simulink model "ModeloCorrea_Cinematico"  (R2023b)
settings: Solver=ode23  StartTime=0.0  StopTime=30  RelTol=1e-3
PreLoadFcn:
  | cargar_datos
model workspace: external: MATLAB File Data\Ensamblaje_Correa_v2_DataFile.m (data not in the file)
undefined symbols (not defined in the file): D, DiscIntNeverNeededParam, Floor, L, R, smiData, X, Y, Z
libraries: sm_lib x464, nesl_utility x23, simulink x8, fl_lib x8, SignalEditorBlockLib x1
(part 1 of 10)
settings Model: Creator=marco  LastModifiedBy=pablo
settings ExplorerConfigSet: InternalSimMechanicsExplorerSettings="<ExplorerConfiguration><canonicalview>default</canonicalview><AnimationSetting><BasePlaybackSpeed>1.0</BasePlaybackSpeed><PlaybackSpeedFactor>1.0</PlaybackSpeedFactor></AnimationSetting><TilePanel><TileInfo><Tiles Columns=\"1\" Count=\"1\" Rows=\"1\"><Column Weight=\"1\"/><Row Weight=\"1\"/><Tile Height=\"1\" Width=\"1\" X=\"0\" Y=\"0\"/></Tiles></TileInfo><SceneInfo><SceneViewer><BGColor><R>0.60000002384185791</R><G>0.60000002384185791</G><B>0.60000002384185791</B></BGColor><Camera><DoPerspective>on</DoPerspective><Position><X>3.93456182089521178</X><Y>0.00766523810611929868</Y><Z>0.735437752381419729</Z></Position><Center><X>3.922559944947976</X><Y>1.61665270142100193</Y><Z>0.0943330044117247912</Z></Center><Up><X>-0.155681862139708971</X><Y>-0.2409665214320105</Y><Z>0.957965705727333972</Z></Up><ViewLimDist>1</ViewLimDist><YLim>0.466307658154998583</YLim><XLim>0.725911711539609095</XLim></Camera></SceneViewer></SceneInfo></TilePanel><MechEditorPanel><Cameras><Camera><Id>Camera1</Id><Value><Name>Camera Esquina</Name><NativeCamera><PositionTrackingFeature>Camaras.Camara_Esquina_Posicion.R</PositionTrackingFeature><CenterTrackingFeature>Camaras.Camara_Aim.R</CenterTrackingFeature><UpVectorTrackingFeature>Camaras.Camara_Esquina_Transformacion.B</UpVectorTrackingFeature><CenterTrackingOrigin>on</CenterTrackingOrigin><UpVectorTrackingDirection>+Z</UpVectorTrackingDirection></NativeCamera></Value></Camera><Camera><Id>Camera2</Id><Value><Name>Camera Lateral</Name><NativeCamera><PositionTrackingFeature>Camaras.Camara_Lateral_Posicion.R</PositionTrackingFeature><CenterTrackingFeature>Camaras.Camara_Aim.R</CenterTrackingFeature><UpVectorTrackingFeature>Camaras.Camara_Lateral_Transformacion.B</UpVectorTrackingFeature><CenterTrackingOrigin>on</CenterTrackingOrigin><UpVectorTrackingDirection>-Y</UpVectorTrackingDirection></NativeCamera></Value></Camera><Camera><Id>Camera3</Id><Value><Name>Camera Superior</Name><NativeCamera><PositionTrackingFeature>Camara_Sup.Camara_Superior_Posicion.R</PositionTrackingFeature><CenterTrackingFeature>Camara_Sup.Camara_Aim.R</CenterTrackingFeature><UpVectorTrackingFeature>Camara_Sup.Camara_Superior_Transformacion.F</UpVectorTrackingFeature><CenterTrackingOrigin>on</CenterTrackingOrigin><UpVectorTrackingDirection>+X</UpVectorTrackingDirection></NativeCamera></Value></Camera></Cameras><GfxPanelCameraMap><MapElement CameraMLId=\"Camera1\" GfxPanelIndex=\"0\"/></GfxPanelCameraMap><VideoCreator><PlaybackSpeedRatio>1.0</PlaybackSpeedRatio><FrameRate>30</FrameRate><VideoFormat>Motion JPEG AVI</VideoFormat><FrameSize>auto</FrameSize></VideoCreator></MechEditorPanel></ExplorerConfiguration>"

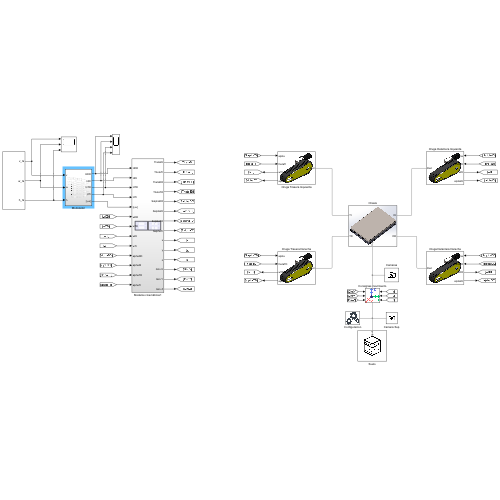
[thumbnail: Simulink's stored preview of the top-level diagram]
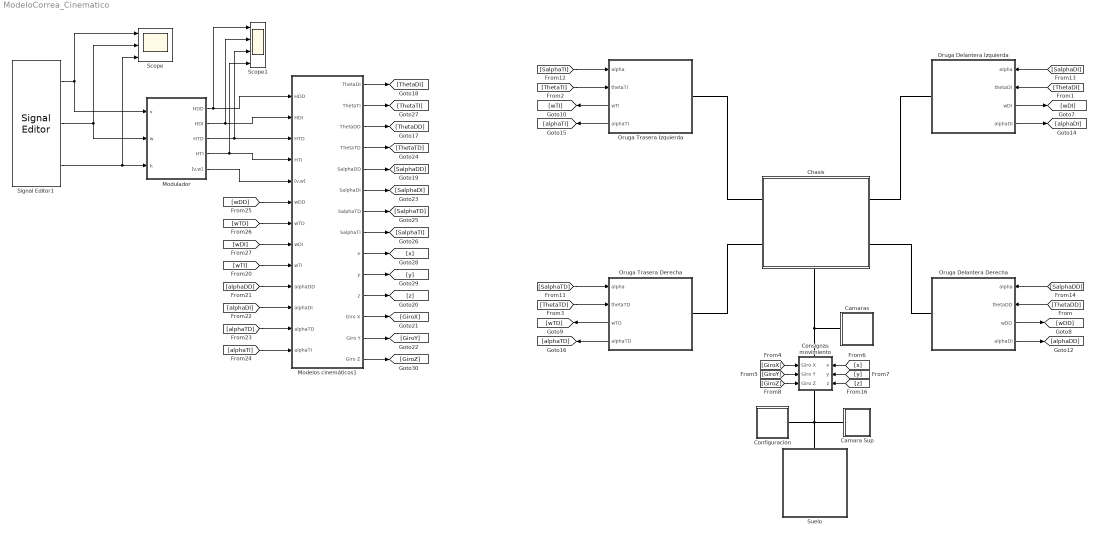
== system ModeloCorrea_Cinematico ==
  Camara Sup : Subsystem
      mask Display: image('photo-camera-icons-photo-camera-icon-design-illustration-photo-camera-simple-sign-photo-camera-logo-free-vector.jpg');
  Camaras : Subsystem
      mask Display: image('photo-camera-icons-photo-camera-icon-design-illustration-photo-camera-simple-sign-photo-camera-logo-free-vector.jpg');
  Chasis : Subsystem
      settings: PortSchema="{\"entries\":[{\"content\":{\"sides\":[{\"content\":{\"connectorIds\":[\"LConn1\",\"LConn2\"]},\"type\":\"ConnectorPlacement.EquallySpacedRectSide\",\"uuid\":\"efc86758-44be-4031-b1cd-a76dbd4a2ab2\"},{\"content\":{\"connectorIds\":[\"RConn1\",\"RConn2\"],\"side\":\"RIGHT\"},\"type\":\"ConnectorPlacement.EquallySpacedRectSide\",\"uuid\":\"c3a2d335-83d2-4f11-a82e-84212a5c33ba\"},{\"content\":{\"side\":\"TOP\"},\"type\":\"ConnectorPlacement.EquallySpacedRectSide\",\"uuid\":\"ad9cdccb-a03b-4b4d-9ef0-e37d712b26c8\"},{\"content\":{\"connectorIds\":[\"RConn3\"],\"side\":\"BOTTOM\"},\"type\":\"ConnectorPlacement.EquallySpacedRectSide\",\"uuid\":\"f3b898e7-922a-430d-876f-1d341c160358\"}]},\"type\":\"ConnectorPlacement.EquallySpacedConnector\",\"uuid\":\"67201c38-8ca0-49d9-b554-1a10d9afc937\"}],\"packageUris\":[\"http://schema.mathworks.com/mf0/Connector/R2020b\"],\"version\":\"1.0\"}"
      mask Display: image('Chasis.png');
  Configuracion : Subsystem
      mask Display: image('config_logo.png');
  Consignas movimiento : Subsystem
      settings: PortSchema="{\"entries\":[{\"content\":{\"sides\":[{\"content\":{\"connectorIds\":[\"In1\",\"In2\",\"In3\"]},\"type\":\"ConnectorPlacement.EquallySpacedRectSide\",\"uuid\":\"6f4dacc9-91b7-4b7c-adf8-17f8e72d409f\"},{\"content\":{\"connectorIds\":[\"In4\",\"In5\",\"In6\"],\"side\":\"RIGHT\"},\"type\":\"ConnectorPlacement.EquallySpacedRectSide\",\"uuid\":\"4738979a-9217-40ad-89d7-912983be4ece\"},{\"content\":{\"connectorIds\":[\"LConn1\"],\"side\":\"TOP\"},\"type\":\"ConnectorPlacement.EquallySpacedRectSide\",\"uuid\":\"3e71380e-8ac2-4639-a71e-f5923b7fda65\"},{\"content\":{\"connectorIds\":[\"RConn1\"],\"side\":\"BOTTOM\"},\"type\":\"ConnectorPlacement.EquallySpacedRectSide\",\"uuid\":\"b318c422-65a3-475f-9e06-26d8c5a1eab3\"}]},\"type\":\"ConnectorPlacement.EquallySpacedConnector\",\"uuid\":\"e032681b-f25a-4d65-b739-2911fc3b0713\"}],\"packageUris\":[\"http://schema.mathworks.com/mf0/Connector/R2020b\"],\"version\":\"1.0\"}"
      mask Display: image('12056247.png');
  Modelos cinemáticos1 : Subsystem
  Modulador : Subsystem
  Oruga Delantera Derecha : Subsystem
      settings: PortSchema="{\"entries\":[{\"content\":{\"sides\":[{\"content\":{\"connectorIds\":[\"LConn1\"]},\"type\":\"ConnectorPlacement.EquallySpacedRectSide\",\"uuid\":\"a1295ca0-b7c0-436a-88be-cceedf21e517\"},{\"content\":{\"connectorIds\":[\"In1\",\"In2\",\"Out1\",\"Out2\"],\"side\":\"RIGHT\"},\"type\":\"ConnectorPlacement.EquallySpacedRectSide\",\"uuid\":\"ea9eb1ac-1c17-440b-aac3-8fa76cfe55ec\"},{\"content\":{\"side\":\"TOP\"},\"type\":\"ConnectorPlacement.EquallySpacedRectSide\",\"uuid\":\"ea9ec6ca-5cdc-41ac-8d7c-823a8b28d2a6\"}]},\"type\":\"ConnectorPlacement.EquallySpacedConnector\",\"uuid\":\"e0ebff2e-a023-4859-a608-17c2594749b2\"}],\"packageUris\":[\"http://schema.mathworks.com/mf0/Connector/R2020b\"],\"version\":\"1.0\"}"
      mask Display: image('OrugaCompleta_Correa.png');
  Oruga Delantera Izquierda : Subsystem
      settings: PortSchema="{\"entries\":[{\"content\":{\"sides\":[{\"content\":{\"connectorIds\":[\"LConn1\"]},\"type\":\"ConnectorPlacement.EquallySpacedRectSide\",\"uuid\":\"a1295ca0-b7c0-436a-88be-cceedf21e517\"},{\"content\":{\"connectorIds\":[\"In1\",\"In2\",\"Out1\",\"Out2\"],\"side\":\"RIGHT\"},\"type\":\"ConnectorPlacement.EquallySpacedRectSide\",\"uuid\":\"ea9eb1ac-1c17-440b-aac3-8fa76cfe55ec\"},{\"content\":{\"side\":\"TOP\"},\"type\":\"ConnectorPlacement.EquallySpacedRectSide\",\"uuid\":\"ea9ec6ca-5cdc-41ac-8d7c-823a8b28d2a6\"}]},\"type\":\"ConnectorPlacement.EquallySpacedConnector\",\"uuid\":\"e0ebff2e-a023-4859-a608-17c2594749b2\"}],\"packageUris\":[\"http://schema.mathworks.com/mf0/Connector/R2020b\"],\"version\":\"1.0\"}"
      mask Display: image('OrugaCompleta_Correa.png');
  Oruga Trasera Derecha : Subsystem
      settings: PortSchema="{\"entries\":[{\"content\":{\"sides\":[{\"content\":{\"connectorIds\":[\"LConn1\"]},\"type\":\"ConnectorPlacement.EquallySpacedRectSide\",\"uuid\":\"a1295ca0-b7c0-436a-88be-cceedf21e517\"},{\"content\":{\"connectorIds\":[\"In1\",\"In2\",\"Out1\",\"Out2\"],\"side\":\"RIGHT\"},\"type\":\"ConnectorPlacement.EquallySpacedRectSide\",\"uuid\":\"ea9eb1ac-1c17-440b-aac3-8fa76cfe55ec\"},{\"content\":{\"side\":\"TOP\"},\"type\":\"ConnectorPlacement.EquallySpacedRectSide\",\"uuid\":\"ea9ec6ca-5cdc-41ac-8d7c-823a8b28d2a6\"}]},\"type\":\"ConnectorPlacement.EquallySpacedConnector\",\"uuid\":\"e0ebff2e-a023-4859-a608-17c2594749b2\"}],\"packageUris\":[\"http://schema.mathworks.com/mf0/Connector/R2020b\"],\"version\":\"1.0\"}"
      mask Display: image('OrugaCompleta_Correa.png');
  Oruga Trasera Izquierda : Subsystem
      settings: PortSchema="{\"entries\":[{\"content\":{\"sides\":[{\"content\":{\"connectorIds\":[\"LConn1\"]},\"type\":\"ConnectorPlacement.EquallySpacedRectSide\",\"uuid\":\"a1295ca0-b7c0-436a-88be-cceedf21e517\"},{\"content\":{\"connectorIds\":[\"In1\",\"In2\",\"Out1\",\"Out2\"],\"side\":\"RIGHT\"},\"type\":\"ConnectorPlacement.EquallySpacedRectSide\",\"uuid\":\"ea9eb1ac-1c17-440b-aac3-8fa76cfe55ec\"},{\"content\":{\"side\":\"TOP\"},\"type\":\"ConnectorPlacement.EquallySpacedRectSide\",\"uuid\":\"ea9ec6ca-5cdc-41ac-8d7c-823a8b28d2a6\"}]},\"type\":\"ConnectorPlacement.EquallySpacedConnector\",\"uuid\":\"e0ebff2e-a023-4859-a608-17c2594749b2\"}],\"packageUris\":[\"http://schema.mathworks.com/mf0/Connector/R2020b\"],\"version\":\"1.0\"}"
      mask Display: image('OrugaCompleta_Correa.png');
  Scope : Scope  NumInputPorts=3
  Scope1 : Scope  NumInputPorts=4
  Signal Editor1 : SignalEditorBlockLib/Signal Editor  FileName=datos_modelo.mat  ActiveScenario=modelo  ActiveSignal=v_ts  IsBus=off  OutputBusObjectStr=Bus: BusObject  SampleTime=0.1  ZeroCross=off  OutputAfterFinalValue=Setting to zero  Unit=inherit  PreserveSignalName=on  ApplySigPropsToAllScenarios=on  ApplySigPropsToAllSignals=on
  Suelo : Subsystem
      mask Display: image('suelo_icon.jpg');
  wires:
  [ThetaDD] -> Oruga Delantera Derecha/2(thetaDD)
  [ThetaDI] -> Oruga Delantera Izquierda/2(thetaDI)
  [ThetaTI] -> Oruga Trasera Izquierda/2(thetaTI)
  [ThetaTD] -> Oruga Trasera Derecha/2(thetaTD)
  Oruga Delantera Izquierda/1(wDI) -> [wDI]
  Oruga Delantera Derecha/1(wDD) -> [wDD]
  Oruga Trasera Derecha/1(wTD) -> [wTD]
  Oruga Trasera Izquierda/1(wTI) -> [wTI]
  [SalphaTD] -> Oruga Trasera Derecha/1(alpha)
  [SalphaTI] -> Oruga Trasera Izquierda/1(alpha)
  [SalphaDI] -> Oruga Delantera Izquierda/1(alpha)
  [SalphaDD] -> Oruga Delantera Derecha/1(alpha)
  Oruga Delantera Derecha/2(alphaDI) -> [alphaDD]
  Oruga Delantera Izquierda/2(alphaDI) -> [alphaDI]
  Oruga Trasera Izquierda/2(alphaTI) -> [alphaTI]
  Oruga Trasera Derecha/2(alphaTD) -> [alphaTD]
  Modelos cinemáticos1/2(ThetaTI) -> [ThetaTI]
  Modelos cinemáticos1/8(SalphaTI) -> [SalphaTI]
  Modelos cinemáticos1/7(SalphaTD) -> [SalphaTD]
  Modelos cinemáticos1/6(SalphaDI) -> [SalphaDI]
  [wDI] -> Modelos cinemáticos1/8(wDI)
  Modelos cinemáticos1/1(ThetaDI) -> [ThetaDI]
  Modelos cinemáticos1/3(ThetaDD) -> [ThetaDD]
  [alphaTI] -> Modelos cinemáticos1/13(alphaTI)
  Modelos cinemáticos1/5(SalphaDD) -> [SalphaDD]
  Modelos cinemáticos1/4(ThetaTD) -> [ThetaTD]
  Modelos cinemáticos1/10(y) -> [y]
  Modelos cinemáticos1/12(Giro X) -> [GiroX]
  [alphaTD] -> Modelos cinemáticos1/12(alphaTD)
  [alphaDI] -> Modelos cinemáticos1/11(alphaDI)
  Modelos cinemáticos1/9(x) -> [x]
  [alphaDD] -> Modelos cinemáticos1/10(alphaDD)
  [wTI] -> Modelos cinemáticos1/9(wTI)
  [wDD] -> Modelos cinemáticos1/6(wDD)
  Modelos cinemáticos1/14(Giro Z) -> [GiroZ]
  [wTD] -> Modelos cinemáticos1/7(wTD)
  Modelos cinemáticos1/11(z) -> [z]
  Modelos cinemáticos1/13(Giro Y) -> [GiroY]
  [GiroZ] -> Consignas movimiento/3(Giro Z)
  [x] -> Consignas movimiento/4(x)
  [GiroY] -> Consignas movimiento/2(Giro Y)
  [GiroX] -> Consignas movimiento/1(Giro X)
  [z] -> Consignas movimiento/6(z)
  [y] -> Consignas movimiento/5(y)
  Signal Editor1/2 -> Scope/2, Modulador/2(w)
  Signal Editor1/1 -> Scope/1, Modulador/1(v)
  Modulador/1(HDD) -> Scope1/1, Modelos cinemáticos1/1(HDD)
  Modulador/2(HDI) -> Scope1/2, Modelos cinemáticos1/2(HDI)
  Modulador/3(HTD) -> Scope1/3, Modelos cinemáticos1/3(HTD)
  Modulador/4(HTI) -> Modelos cinemáticos1/4(HTI), Scope1/4
  Modulador/5("[v,w]") -> Modelos cinemáticos1/5("[v,w]")
  Signal Editor1/3 -> Modulador/3(h), Scope/3
  connections:
  Suelo/LConn1 -- Camara Sup/RConn1 -- Consignas movimiento/RConn1 -- Configuracion/RConn1
  Chasis/LConn2 -- Oruga Trasera Derecha/LConn1
  Chasis/LConn1 -- Oruga Trasera Izquierda/LConn1
  Chasis/RConn1 -- Oruga Delantera Izquierda/LConn1
  Chasis/RConn2 -- Oruga Delantera Derecha/LConn1
  Camaras/RConn1 -- Chasis/RConn3 -- Consignas movimiento/LConn1

== system ModeloCorrea_Cinematico/Camara Sup ==
  Camara Aim : sm_lib/Frames and Transforms/Reference Frame
  Camara Superior Posicion : sm_lib/Frames and Transforms/Reference Frame
  Camara Superior Transformacion : sm_lib/Frames and Transforms/Rigid Transform  TranslationMethod=Cartesian  TranslationStandardOffset=0  TranslationStandardOffsetUnits=m  TranslationStandardAxis=+Z  TranslationCartesianOffset=[0 0 -10]  TranslationCartesianOffsetUnits=m  TranslationROffset=0  TranslationROffsetUnits=m  TranslationZOffset=0  TranslationZOffsetUnits=m  TranslationThetaOffset=0  TranslationThetaOffsetUnits=deg  RotationMethod=None  RotationAngleUnits=deg  RotationStandardAxis=+Z  RotationAngle=0.0  RotationArbitraryAxis=[0 0 1]  FollAlignAxisA=+X  BaseAlignAxisA=+Y  FollAlignAxisB=+Y  BaseAlignAxisB=+Z  RotationSequenceAxes=FollowerAxes  RotationSequence=XYX  RotationSequenceAngles=[0 0 0]  RotationSequenceAnglesUnits=deg  RotationMatrix=[1 0 0; 0 1 0; 0 0 1]  Quaternion=[1 0 0 0]
  Camara Superior : PMIOPort  Side=Right
  connections:
  Camara Superior Posicion/RConn1 -- Camara Superior Transformacion/LConn1
  Camara Aim/RConn1 -- Camara Superior Transformacion/RConn1 -- Camara Superior/RConn1

== system ModeloCorrea_Cinematico/Camaras ==
  Camara Aim : sm_lib/Frames and Transforms/Reference Frame
  Camara Esquina Posicion : sm_lib/Frames and Transforms/Reference Frame
  Camara Esquina Transformacion : sm_lib/Frames and Transforms/Rigid Transform  TranslationMethod=Cartesian  TranslationStandardOffset=0  TranslationStandardOffsetUnits=m  TranslationStandardAxis=+Z  TranslationCartesianOffset=[-1 -1 -1]  TranslationCartesianOffsetUnits=m  TranslationROffset=0  TranslationROffsetUnits=m  TranslationZOffset=0  TranslationZOffsetUnits=m  TranslationThetaOffset=0  TranslationThetaOffsetUnits=deg  RotationMethod=None  RotationAngleUnits=deg  RotationStandardAxis=+Z  RotationAngle=0.0  RotationArbitraryAxis=[0 0 1]  FollAlignAxisA=+X  BaseAlignAxisA=+Y  FollAlignAxisB=+Y  BaseAlignAxisB=+Z  RotationSequenceAxes=FollowerAxes  RotationSequence=XYX  RotationSequenceAngles=[0 0 0]  RotationSequenceAnglesUnits=deg  RotationMatrix=[1 0 0; 0 1 0; 0 0 1]  Quaternion=[1 0 0 0]
  Camara Lateral Posicion : sm_lib/Frames and Transforms/Reference Frame
  Camara Lateral Transformacion : sm_lib/Frames and Transforms/Rigid Transform  TranslationMethod=Cartesian  TranslationStandardOffset=0  TranslationStandardOffsetUnits=m  TranslationStandardAxis=+Z  TranslationCartesianOffset=[0 -2 -0.30]  TranslationCartesianOffsetUnits=m  TranslationROffset=0  TranslationROffsetUnits=m  TranslationZOffset=0  TranslationZOffsetUnits=m  TranslationThetaOffset=0  TranslationThetaOffsetUnits=deg  RotationMethod=None  RotationAngleUnits=deg  RotationStandardAxis=+Z  RotationAngle=0.0  RotationArbitraryAxis=[0 0 1]  FollAlignAxisA=+X  BaseAlignAxisA=+Y  FollAlignAxisB=+Y  BaseAlignAxisB=+Z  RotationSequenceAxes=FollowerAxes  RotationSequence=XYX  RotationSequenceAngles=[0 0 0]  RotationSequenceAnglesUnits=deg  RotationMatrix=[1 0 0; 0 1 0; 0 0 1]  Quaternion=[1 0 0 0]
  Camaras : PMIOPort  Side=Right
  connections:
  Camara Esquina Transformacion/RConn1 -- Camara Lateral Transformacion/RConn1 -- Camara Aim/RConn1 -- Camaras/RConn1
  Camara Esquina Posicion/RConn1 -- Camara Esquina Transformacion/LConn1
  Camara Lateral Posicion/RConn1 -- Camara Lateral Transformacion/LConn1

== system ModeloCorrea_Cinematico/Chasis ==
  ReferenceFrame : sm_lib/Frames and Transforms/Reference Frame
  Rigid Transform1 : sm_lib/Frames and Transforms/Rigid Transform  TranslationMethod=Cartesian  TranslationStandardOffset=91.5  TranslationStandardOffsetUnits=mm  TranslationStandardAxis=-X  TranslationCartesianOffset=[91.5 -70 +158.5]  TranslationCartesianOffsetUnits=mm  TranslationROffset=0  TranslationROffsetUnits=m  TranslationZOffset=0  TranslationZOffsetUnits=m  TranslationThetaOffset=0  TranslationThetaOffsetUnits=deg  RotationMethod=StandardAxis  RotationAngleUnits=deg  RotationStandardAxis=+Y  RotationAngle=180  RotationArbitraryAxis=[1 1 0]  FollAlignAxisA=+X  BaseAlignAxisA=+Y  FollAlignAxisB=+Y  BaseAlignAxisB=+Z  RotationSequenceAxes=FollowerAxes  RotationSequence=XYX  RotationSequenceAngles=[180 180 0]  RotationSequenceAnglesUnits=deg  RotationMatrix=[0 180 0; 0 1 0; 0 0 1]  Quaternion=[1 0 0 0]
  Rigid Transform2 : sm_lib/Frames and Transforms/Rigid Transform  TranslationMethod=Cartesian  TranslationStandardOffset=91.5  TranslationStandardOffsetUnits=mm  TranslationStandardAxis=-X  TranslationCartesianOffset=[91.5 -70 -158.5]  TranslationCartesianOffsetUnits=mm  TranslationROffset=0  TranslationROffsetUnits=m  TranslationZOffset=0  TranslationZOffsetUnits=m  TranslationThetaOffset=0  TranslationThetaOffsetUnits=deg  RotationMethod=StandardAxis  RotationAngleUnits=deg  RotationStandardAxis=+Y  RotationAngle=180  RotationArbitraryAxis=[0 0 1]  FollAlignAxisA=+X  BaseAlignAxisA=+Y  FollAlignAxisB=+Y  BaseAlignAxisB=+Z  RotationSequenceAxes=FollowerAxes  RotationSequence=XYX  RotationSequenceAngles=[0 0 0]  RotationSequenceAnglesUnits=deg  RotationMatrix=[1 0 0; 0 1 0; 0 0 1]  Quaternion=[1 0 0 0]
  Rigid Transform3 : sm_lib/Frames and Transforms/Rigid Transform  TranslationMethod=Cartesian  TranslationStandardOffset=91.5  TranslationStandardOffsetUnits=mm  TranslationStandardAxis=-X  TranslationCartesianOffset=[-91.5 -70 -158.5]  TranslationCartesianOffsetUnits=mm  TranslationROffset=0  TranslationROffsetUnits=m  TranslationZOffset=0  TranslationZOffsetUnits=m  TranslationThetaOffset=0  TranslationThetaOffsetUnits=deg  RotationMethod=None  RotationAngleUnits=deg  RotationStandardAxis=+X  RotationAngle=180  RotationArbitraryAxis=[1 1 0]  FollAlignAxisA=+X  BaseAlignAxisA=+Y  FollAlignAxisB=+Y  BaseAlignAxisB=+Z  RotationSequenceAxes=FollowerAxes  RotationSequence=XYX  RotationSequenceAngles=[180 180 0]  RotationSequenceAnglesUnits=deg  RotationMatrix=[0 180 0; 0 1 0; 0 0 1]  Quaternion=[1 0 0 0]
  Rigid Transform4 : sm_lib/Frames and Transforms/Rigid Transform  TranslationMethod=Cartesian  TranslationStandardOffset=91.5  TranslationStandardOffsetUnits=mm  TranslationStandardAxis=-X  TranslationCartesianOffset=[-91.5 -70 158.5]  TranslationCartesianOffsetUnits=mm  TranslationROffset=0  TranslationROffsetUnits=m  TranslationZOffset=0  TranslationZOffsetUnits=m  TranslationThetaOffset=0  TranslationThetaOffsetUnits=deg  RotationMethod=None  RotationAngleUnits=deg  RotationStandardAxis=+Z  RotationAngle=0.0  RotationArbitraryAxis=[0 0 1]  FollAlignAxisA=+X  BaseAlignAxisA=+Y  FollAlignAxisB=+Y  BaseAlignAxisB=+Z  RotationSequenceAxes=FollowerAxes  RotationSequence=XYX  RotationSequenceAngles=[0 0 0]  RotationSequenceAnglesUnits=deg  RotationMatrix=[1 0 0; 0 1 0; 0 0 1]  Quaternion=[1 0 0 0]
  Rigid Transform5 : sm_lib/Frames and Transforms/Rigid Transform  TranslationMethod=StandardAxis  TranslationStandardOffset=235  TranslationStandardOffsetUnits=mm  TranslationStandardAxis=+Z  TranslationCartesianOffset=[0 0 0]  TranslationCartesianOffsetUnits=m  TranslationROffset=0  TranslationROffsetUnits=m  TranslationZOffset=0  TranslationZOffsetUnits=m  TranslationThetaOffset=0  TranslationThetaOffsetUnits=deg  RotationMethod=StandardAxis  RotationAngleUnits=deg  RotationStandardAxis=+X  RotationAngle=90  RotationArbitraryAxis=[0 0 1]  FollAlignAxisA=+X  BaseAlignAxisA=+Y  FollAlignAxisB=+Y  BaseAlignAxisB=+Z  RotationSequenceAxes=FollowerAxes  RotationSequence=XYX  RotationSequenceAngles=[0 0 0]  RotationSequenceAnglesUnits=deg  RotationMatrix=[1 0 0; 0 1 0; 0 0 1]  Quaternion=[1 0 0 0]
  Solid : sm_lib/Body Elements/File Solid  ExtGeomFileName=CAD\Chasis.STEP  UnitType=FromFile  ExtGeomFileUnits=m  StepReaderType=HEX  ExportConvexHullGeometry=off  InertiaType=Custom  Mass=100  MassUnits=kg  CenterOfMass=smiData.Solid(19).CoM  CenterOfMassUnits=mm  MomentsOfInertia=smiData.Solid(19).MoI  MomentsOfInertiaUnits=kg*mm^2  ProductsOfInertia=smiData.Solid(19).PoI  ProductsOfInertiaUnits=kg*mm^2  BasedOnType=DensityFromFile  Density=1000  DensityUnits=kg/m^3  DoExposeReferenceFrame=on  SerializedFrames=<Frames/>  GraphicType=FromGeometry  MarkerShape=Sphere  MarkerSize=10  GraphicVisPropType=SimpleVisualProperties  GraphicDiffuseColor=[0.6 0.6 0.6]  GraphicSpecularColor=[0.5 0.5 0.5 1.0]  GraphicAmbientColor=[0.15 0.15 0.15 1.0]  GraphicEmissiveColor=[0.0 0.0 0.0 1.0]  GraphicShininess=75  GraphicOpacity=smiData.Solid(19).opacity
  TI : PMIOPort  Side=Left
  TD : PMIOPort  Port=2  Side=Left
  DI : PMIOPort  Port=3  Side=Right
  DD : PMIOPort  Port=4  Side=Right
  Input : PMIOPort  Port=5  Side=Right
  connections:
  Rigid Transform5/LConn1 -- Input/RConn1
  TD/RConn1 -- Rigid Transform4/RConn1
  Rigid Transform3/LConn1 -- Rigid Transform2/LConn1 -- Solid/RConn1 -- Rigid Transform1/LConn1 -- Rigid Transform5/RConn1 -- Rigid Transform4/LConn1 -- ReferenceFrame/RConn1
  Rigid Transform3/RConn1 -- TI/RConn1
  DI/RConn1 -- Rigid Transform2/RConn1
  Rigid Transform1/RConn1 -- DD/RConn1

== system ModeloCorrea_Cinematico/Configuracion ==
  MechanismConfiguration : sm_lib/Utilities/Mechanism Configuration  UniformGravity=Constant  GravityVector=[0 -9.80665 0]  GravityVectorUnits=m/s^2  LinearizationDelta=0.001  JointModeTransitionNonlinearIterations=2
  Solver Configuration : nesl_utility/Solver Configuration  PhysicalDomain=network_engine_domain  SubClassName=solver  LeftPortType=input  RightPortType=generic  Tones=[]  Harmonics=[]  SimulateNoise=off  Profile=off  UseLocalSampling=off  EnableSwitchedLinearOptims=on  FrequencyDomain=off  UseCCode=off  RelTol=0.001  AbsTol=0.001  MinStep=1e-09  ToWorkspace=off  RevertToSquareIcSolve=off  NumHomotopyIterations=100  PhasorMode=off  PhasorModeNumHarmonics=1  ConsistencySolver=NEWTON_XTOL_AFTER_FTOL  IndexReductionMethod=DerivativeReplacement  DoDC=off  ResidualTolerance=1e-09  ConsistencyTolSource=GLOBAL  ConsistencyAbsTol=0.001  ConsistencyRelTol=0.001  ConsistencyTolFactor=0.001  UseLocalSolver=off  LocalSolverChoice=NE_BACKWARD_EULER_ADVANCER  ResolveIndetEquations=on  FunctionEvalNumThread=1  LocalSolverSampleTime=0.001  DoFixedCost=off  MaxNonlinIter=3  MaxModeIter=2  ComputeImpulses=off  ImpulseIterations=2  LinearAlgebra=auto  LinearAlgebraNumThread=0  EquationFormulation=NE_TIME_EF  DelaysMemoryBudget=1024  AutomaticFiltering=on  FilteringTimeConstant=0.001  PartitionStorageMethod=AS_NEEDED  PartitionMemoryBudget=1024  PartitionMethod=ROBUST  MultibodyUseLocalSolver=off  MultibodyLocalSolverChoice=ODE1  MultibodyLocalSolverSampleTime=0.001
  World : sm_lib/Frames and Transforms/World Frame
  a : PMIOPort  Side=Right
  connections:
  World/RConn1 -- MechanismConfiguration/RConn1 -- Solver Configuration/RConn1 -- a/RConn1

== system ModeloCorrea_Cinematico/Consignas movimiento ==
  Giro X : Inport
  Giro Y : Inport  Port=2
  Giro Z : Inport  Port=3
  x : Inport  Port=4
  y : Inport  Port=5
  z : Inport  Port=6
  Bushing Joint : sm_lib/Joints/Bushing Joint  JointMode=Normal  SenseConstraintForce=off  SenseConstraintForceX=off  SenseConstraintForceY=off  SenseConstraintForceZ=off  SenseConstraintTorque=off  SenseConstraintTorqueX=off  SenseConstraintTorqueY=off  SenseConstraintTorqueZ=off  SenseTotalForce=off  SenseTotalForceX=off  SenseTotalForceY=off  SenseTotalForceZ=off  SenseTotalTorque=off  SenseTotalTorqueX=off  SenseTotalTorqueY=off  SenseTotalTorqueZ=off  CompositeWrenchDir=BaseOnFollower  CompositeWrenchFrame=BaseFrame  PxEquilibriumPosition=0  PxEquilibriumPositionUnits=m  PxSpringStiffness=0  PxSpringStiffnessUnits=N/m  PxDampingCoefficient=0  PxDampingCoefficientUnits=N/(m/s)  PxTorqueActuationMode=ComputedTorque  PxMotionActuationMode=InputMotion  PxSensePosition=off  PxSenseVelocity=off  PxSenseAcceleration=off  PxSenseTorqueForce=off  PxSenseLowerLimitTorqueForce=off  PxSenseUpperLimitTorqueForce=off  PxLowerLimitSpecify=off  PxLowerLimitBound=-1  PxLowerLimitBoundUnits=m  PxLowerLimitStiffness=1e6  PxLowerLimitStiffnessUnits=N/m  PxLowerLimitDamping=1e3  PxLowerLimitDampingUnits=N/(m/s)  PxLowerLimitTransitionRegionWidth=1e-4  PxLowerLimitTransitionRegionWidthUnits=m  PxUpperLimitSpecify=off  PxUpperLimitBound=1  PxUpperLimitBoundUnits=m  PxUpperLimitStiffness=1e6  PxUpperLimitStiffnessUnits=N/m  PxUpperLimitDamping=1e3  PxUpperLimitDampingUnits=N/(m/s)  PxUpperLimitTransitionRegionWidth=1e-4  PxUpperLimitTransitionRegionWidthUnits=m  PxPositionTargetSpecify=off  PxPositionTargetPriority=High  PxPositionTargetValue=0  PxPositionTargetValueUnits=m  PxVelocityTargetSpecify=off  PxVelocityTargetPriority=High  PxVelocityTargetValue=0  PxVelocityTargetValueUnits=m/s  PyEquilibriumPosition=0  PyEquilibriumPositionUnits=m  PySpringStiffness=0  PySpringStiffnessUnits=N/m  PyDampingCoefficient=0  PyDampingCoefficientUnits=N/(m/s)  PyTorqueActuationMode=ComputedTorque  PyMotionActuationMode=InputMotion  PySensePosition=off  PySenseVelocity=off  PySenseAcceleration=off  PySenseTorqueForce=off  PySenseLowerLimitTorqueForce=off  PySenseUpperLimitTorqueForce=off  PyLowerLimitSpecify=off  PyLowerLimitBound=-1  PyLowerLimitBoundUnits=m  PyLowerLimitStiffness=1e6  PyLowerLimitStiffnessUnits=N/m  PyLowerLimitDamping=1e3  PyLowerLimitDampingUnits=N/(m/s)  PyLowerLimitTransitionRegionWidth=1e-4  PyLowerLimitTransitionRegionWidthUnits=m  PyUpperLimitSpecify=off  PyUpperLimitBound=1  PyUpperLimitBoundUnits=m  PyUpperLimitStiffness=1e6  PyUpperLimitStiffnessUnits=N/m  PyUpperLimitDamping=1e3  PyUpperLimitDampingUnits=N/(m/s)  PyUpperLimitTransitionRegionWidth=1e-4  PyUpperLimitTransitionRegionWidthUnits=m  PyPositionTargetSpecify=off  PyPositionTargetPriority=High  PyPositionTargetValue=0  PyPositionTargetValueUnits=m  PyVelocityTargetSpecify=off  PyVelocityTargetPriority=High  PyVelocityTargetValue=0  PyVelocityTargetValueUnits=m/s  PzEquilibriumPosition=0  PzEquilibriumPositionUnits=m  PzSpringStiffness=0  PzSpringStiffnessUnits=N/m  PzDampingCoefficient=0  PzDampingCoefficientUnits=N/(m/s)  PzTorqueActuationMode=ComputedTorque  PzMotionActuationMode=InputMotion  PzSensePosition=off  PzSenseVelocity=off  PzSenseAcceleration=off  PzSenseTorqueForce=off  PzSenseLowerLimitTorqueForce=off  PzSenseUpperLimitTorqueForce=off  PzLowerLimitSpecify=off  PzLowerLimitBound=-1  PzLowerLimitBoundUnits=m  PzLowerLimitStiffness=1e6  PzLowerLimitStiffnessUnits=N/m  PzLowerLimitDamping=1e3  PzLowerLimitDampingUnits=N/(m/s)  PzLowerLimitTransitionRegionWidth=1e-4  PzLowerLimitTransitionRegionWidthUnits=m  PzUpperLimitSpecify=off  PzUpperLimitBound=1  PzUpperLimitBoundUnits=m  PzUpperLimitStiffness=1e6  PzUpperLimitStiffnessUnits=N/m  PzUpperLimitDamping=1e3  PzUpperLimitDampingUnits=N/(m/s)  PzUpperLimitTransitionRegionWidth=1e-4  PzUpperLimitTransitionRegionWidthUnits=m  PzPositionTargetSpecify=off  PzPositionTargetPriority=High  PzPositionTargetValue=0  PzPositionTargetValueUnits=m  PzVelocityTargetSpecify=off  PzVelocityTargetPriority=High  PzVelocityTargetValue=0  PzVelocityTargetValueUnits=m/s  RxEquilibriumPosition=0  RxEquilibriumPositionUnits=deg  RxSpringStiffness=0  RxSpringStiffnessUnits=N*m/deg  RxDampingCoefficient=0  RxDampingCoefficientUnits=N*m/(deg/s)  RxTorqueActuationMode=ComputedTorque  RxMotionActuationMode=InputMotion  RxSensePosition=off  RxSenseVelocity=off  RxSenseAcceleration=off  RxSenseTorqueForce=off  RxSenseLowerLimitTorqueForce=off  RxSenseUpperLimitTorqueForce=off  RxLowerLimitSpecify=off  RxLowerLimitBound=-90  RxLowerLimitBoundUnits=deg  RxLowerLimitStiffness=1e4  RxLowerLimitStiffnessUnits=N*m/deg  RxLowerLimitDamping=10  RxLowerLimitDampingUnits=N*m/(deg/s)  RxLowerLimitTransitionRegionWidth=0.1  RxLowerLimitTransitionRegionWidthUnits=deg  RxUpperLimitSpecify=off  RxUpperLimitBound=90  RxUpperLimitBoundUnits=deg  RxUpperLimitStiffness=1e4  RxUpperLimitStiffnessUnits=N*m/deg  RxUpperLimitDamping=10  RxUpperLimitDampingUnits=N*m/(deg/s)  RxUpperLimitTransitionRegionWidth=0.1  RxUpperLimitTransitionRegionWidthUnits=deg  RxPositionTargetSpecify=off  RxPositionTargetPriority=High  RxPositionTargetValue=0  RxPositionTargetValueUnits=deg  RxVelocityTargetSpecify=off  RxVelocityTargetPriority=High  RxVelocityTargetValue=0  RxVelocityTargetValueUnits=deg/s  RyEquilibriumPosition=0  RyEquilibriumPositionUnits=deg  RySpringStiffness=0  RySpringStiffnessUnits=N*m/deg  RyDampingCoefficient=0  RyDampingCoefficientUnits=N*m/(deg/s)  RyTorqueActuationMode=ComputedTorque  RyMotionActuationMode=InputMotion  RySensePosition=off  RySenseVelocity=off  RySenseAcceleration=off  RySenseTorqueForce=off  RySenseLowerLimitTorqueForce=off  RySenseUpperLimitTorqueForce=off  RyLowerLimitSpecify=off  RyLowerLimitBound=-90  RyLowerLimitBoundUnits=deg  RyLowerLimitStiffness=1e4  RyLowerLimitStiffnessUnits=N*m/deg  RyLowerLimitDamping=10  RyLowerLimitDampingUnits=N*m/(deg/s)  RyLowerLimitTransitionRegionWidth=0.1  RyLowerLimitTransitionRegionWidthUnits=deg  RyUpperLimitSpecify=off  RyUpperLimitBound=90  RyUpperLimitBoundUnits=deg  RyUpperLimitStiffness=1e4  RyUpperLimitStiffnessUnits=N*m/deg  RyUpperLimitDamping=10  RyUpperLimitDampingUnits=N*m/(deg/s)  RyUpperLimitTransitionRegionWidth=0.1  RyUpperLimitTransitionRegionWidthUnits=deg  RyPositionTargetSpecify=off  RyPositionTargetPriority=High  RyPositionTargetValue=0  RyPositionTargetValueUnits=deg  RyVelocityTargetSpecify=off  RyVelocityTargetPriority=High  RyVelocityTargetValue=0  RyVelocityTargetValueUnits=deg/s  RzEquilibriumPosition=0  RzEquilibriumPositionUnits=deg  RzSpringStiffness=0  RzSpringStiffnessUnits=N*m/deg  RzDampingCoefficient=0  RzDampingCoefficientUnits=N*m/(deg/s)  RzTorqueActuationMode=ComputedTorque  RzMotionActuationMode=InputMotion  RzSensePosition=off  RzSenseVelocity=off  RzSenseAcceleration=off  RzSenseTorqueForce=off  RzSenseLowerLimitTorqueForce=off  RzSenseUpperLimitTorqueForce=off  RzLowerLimitSpecify=off  RzLowerLimitBound=-90  RzLowerLimitBoundUnits=deg  RzLowerLimitStiffness=1e4  RzLowerLimitStiffnessUnits=N*m/deg  RzLowerLimitDamping=10  RzLowerLimitDampingUnits=N*m/(deg/s)  RzLowerLimitTransitionRegionWidth=0.1  RzLowerLimitTransitionRegionWidthUnits=deg  RzUpperLimitSpecify=off  RzUpperLimitBound=90  RzUpperLimitBoundUnits=deg  RzUpperLimitStiffness=1e4  RzUpperLimitStiffnessUnits=N*m/deg  RzUpperLimitDamping=10  RzUpperLimitDampingUnits=N*m/(deg/s)  RzUpperLimitTransitionRegionWidth=0.1  RzUpperLimitTransitionRegionWidthUnits=deg  RzPositionTargetSpecify=off  RzPositionTargetPriority=High  RzPositionTargetValue=0  RzPositionTargetValueUnits=deg  RzVelocityTargetSpecify=off  RzVelocityTargetPriority=High  RzVelocityTargetValue=0  RzVelocityTargetValueUnits=deg/s
  Simulink-PS Converter{,1..5} (6 alike) : nesl_utility/Simulink-PS Converter  PhysicalDomain=network_engine_domain  SubClassName=ps_input  LeftPortType=input  RightPortType=output  PseudoPeriodic=off  Frequencies=[]  NoiseDistribution=none  NoiseParameters=[]  Unit=1  AffineConversion=off  FilteringAndDerivatives=filter  SimscapeFilterOrder=2  InputFilterTimeConstant=0.001  UdotUserProvided=0
  Output : PMIOPort  Side=Left
  Input : PMIOPort  Port=2  Side=Right
  wires:
  Giro Z/1 -> Simulink-PS Converter4/1
  x/1 -> Simulink-PS Converter/1
  y/1 -> Simulink-PS Converter1/1
  Giro X/1 -> Simulink-PS Converter3/1
  Giro Y/1 -> Simulink-PS Converter5/1
  z/1 -> Simulink-PS Converter2/1
  connections:
  Bushing Joint/RConn1 -- Output/RConn1
  Bushing Joint/LConn1 -- Input/RConn1
  Simulink-PS Converter/RConn1 -- Bushing Joint/LConn2
  Simulink-PS Converter1/RConn1 -- Bushing Joint/LConn3
  Simulink-PS Converter2/RConn1 -- Bushing Joint/LConn4
  Simulink-PS Converter3/RConn1 -- Bushing Joint/LConn5
  Simulink-PS Converter5/RConn1 -- Bushing Joint/LConn6
  Simulink-PS Converter4/RConn1 -- Bushing Joint/LConn7

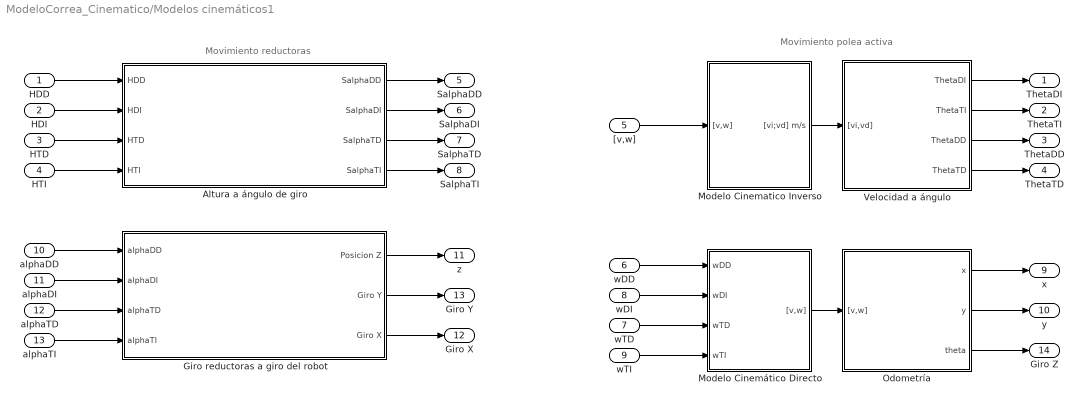
== system ModeloCorrea_Cinematico/Modelos cinemáticos1 ==
  note: Movimiento polea activa
  note: Movimiento reductoras
  HDD : Inport
  HDI : Inport  Port=2
  HTD : Inport  Port=3
  HTI : Inport  Port=4
  "[v,w]" : Inport  Port=5
  wDD : Inport  Port=6
  wTD : Inport  Port=7
  wDI : Inport  Port=8
  wTI : Inport  Port=9
  alphaDD : Inport  Port=10
  alphaDI : Inport  Port=11
  alphaTD : Inport  Port=12
  alphaTI : Inport  Port=13
  Altura a ángulo de giro : Subsystem
  Giro reductoras a giro del robot : Subsystem
  Modelo Cinematico Inverso : Subsystem
  Modelo Cinemático Directo : Subsystem
  Odometría : Subsystem
  Velocidad a ángulo : Subsystem
  ThetaDI : Outport
  ThetaTI : Outport  Port=2
  ThetaDD : Outport  Port=3
  ThetaTD : Outport  Port=4
  SalphaDD : Outport  Port=5
  SalphaDI : Outport  Port=6
  SalphaTD : Outport  Port=7
  SalphaTI : Outport  Port=8
  x : Outport  Port=9
  y : Outport  Port=10
  z : Outport  Port=11
  Giro X : Outport  Port=12
  Giro Y : Outport  Port=13
  Giro Z : Outport  Port=14
  wires:
  alphaDD/1 -> Giro reductoras a giro del robot/1(alphaDD)
  alphaTI/1 -> Giro reductoras a giro del robot/4(alphaTI)
  alphaTD/1 -> Giro reductoras a giro del robot/3(alphaTD)
  alphaDI/1 -> Giro reductoras a giro del robot/2(alphaDI)
  Giro reductoras a giro del robot/1(Posicion Z) -> z/1
  HDD/1 -> Altura a ángulo de giro/1(HDD)
  Altura a ángulo de giro/1(SalphaDD) -> SalphaDD/1
  HTD/1 -> Altura a ángulo de giro/3(HTD)
  HDI/1 -> Altura a ángulo de giro/2(HDI)
  HTI/1 -> Altura a ángulo de giro/4(HTI)
  Altura a ángulo de giro/4(SalphaTI) -> SalphaTI/1
  Altura a ángulo de giro/3(SalphaTD) -> SalphaTD/1
  Altura a ángulo de giro/2(SalphaDI) -> SalphaDI/1
  Giro reductoras a giro del robot/2(Giro Y) -> Giro Y/1
  Giro reductoras a giro del robot/3(Giro X) -> Giro X/1
  Modelo Cinematico Inverso/1("[vi;vd] m/s") -> Velocidad a ángulo/1("[vi,vd]")
  "[v,w]"/1 -> Modelo Cinematico Inverso/1("[v,w]")
  Modelo Cinemático Directo/1("[v,w]") -> Odometría/1("[v,w]")
  wDD/1 -> Modelo Cinemático Directo/1(wDD)
  wDI/1 -> Modelo Cinemático Directo/2(wDI)
  wTD/1 -> Modelo Cinemático Directo/3(wTD)
  wTI/1 -> Modelo Cinemático Directo/4(wTI)
  Velocidad a ángulo/1(ThetaDI) -> ThetaDI/1
  Velocidad a ángulo/2(ThetaTI) -> ThetaTI/1
  Velocidad a ángulo/3(ThetaDD) -> ThetaDD/1
  Velocidad a ángulo/4(ThetaTD) -> ThetaTD/1
  Odometría/1(x) -> x/1
  Odometría/2(y) -> y/1
  Odometría/3(theta) -> Giro Z/1

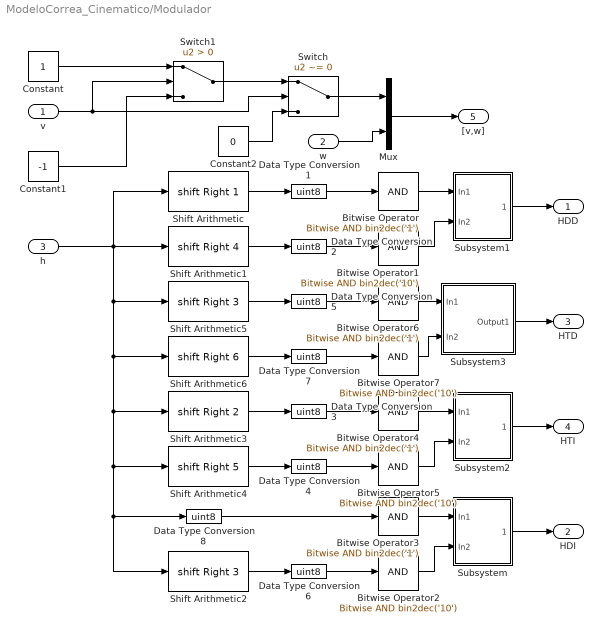
== system ModeloCorrea_Cinematico/Modulador ==
  v : Inport
  w : Inport  Port=2
  h : Inport  Port=3
  Bitwise Operator{,3..4,6} (4 alike) : simulink/Logic and Bit Operations/Bitwise Operator  logicop=AND  UseBitMask=on  BitMask=bin2dec('1')  BitMaskRealWorld=Stored Integer
  Bitwise Operator{1..2,5,7} (4 alike) : simulink/Logic and Bit Operations/Bitwise Operator  logicop=AND  UseBitMask=on  BitMask=bin2dec('10')  BitMaskRealWorld=Stored Integer
  Constant : Constant
  Constant1 : Constant  Value=-1
  Constant2 : Constant  Value=0
  Data Type Conversion{1..8} (8 alike) : DataTypeConversion  OutDataTypeStr=uint8  ConvertRealWorld=Stored Integer (SI)  SaturateOnIntegerOverflow=off  RndMeth=Floor
  Mux : Mux  Inputs=2
  Shift Arithmetic : ArithShift  BitShiftNumber=1  BinPtShiftNumber=8  BitShiftDirection=Right
  Shift Arithmetic1 : ArithShift  BitShiftNumber=4  BinPtShiftNumber=8  BitShiftDirection=Right
  Shift Arithmetic2 : ArithShift  BitShiftNumber=3  BinPtShiftNumber=8  BitShiftDirection=Right
  Shift Arithmetic3 : ArithShift  BitShiftNumber=2  BinPtShiftNumber=8  BitShiftDirection=Right
  Shift Arithmetic4 : ArithShift  BitShiftNumber=5  BinPtShiftNumber=8  BitShiftDirection=Right
  Shift Arithmetic5 : ArithShift  BitShiftNumber=3  BinPtShiftNumber=8  BitShiftDirection=Right
  Shift Arithmetic6 : ArithShift  BitShiftNumber=6  BinPtShiftNumber=8  BitShiftDirection=Right
  Subsystem : Subsystem
  Subsystem1 : Subsystem
  Subsystem2 : Subsystem
  Subsystem3 : Subsystem
  Switch : Switch  Criteria=u2 ~= 0  SaturateOnIntegerOverflow=off  InputSameDT=off
  Switch1 : Switch  Criteria=u2 > Threshold  SaturateOnIntegerOverflow=off  InputSameDT=off
  HDD : Outport
  HDI : Outport  Port=2
  HTD : Outport  Port=3
  HTI : Outport  Port=4
  "[v,w]" : Outport  Port=5
  wires:
  Constant/1 -> Switch1/1
  Constant1/1 -> Switch1/3
  v/1 -> Switch/2, Switch1/2
  Shift Arithmetic/1 -> Data Type Conversion1/1
  h/1 -> Shift Arithmetic2/1, Data Type Conversion8/1, Shift Arithmetic4/1, Shift Arithmetic3/1, Shift Arithmetic6/1, Shift Arithmetic5/1, Shift Arithmetic1/1, Shift Arithmetic/1
  Switch1/1 -> Switch/1
  Constant2/1 -> Switch/3
  Shift Arithmetic1/1 -> Data Type Conversion2/1
  Shift Arithmetic5/1 -> Data Type Conversion5/1
  Shift Arithmetic4/1 -> Data Type Conversion4/1
  Shift Arithmetic6/1 -> Data Type Conversion7/1
  Shift Arithmetic3/1 -> Data Type Conversion3/1
  Data Type Conversion8/1 -> Bitwise Operator3/1
  Shift Arithmetic2/1 -> Data Type Conversion6/1
  Data Type Conversion7/1 -> Bitwise Operator7/1
  Switch/1 -> Mux/1
  w/1 -> Mux/2
  Bitwise Operator1/1 -> Subsystem1/2(In2)
  Data Type Conversion1/1 -> Bitwise Operator/1
  Data Type Conversion2/1 -> Bitwise Operator1/1
  Data Type Conversion5/1 -> Bitwise Operator6/1
  Data Type Conversion4/1 -> Bitwise Operator5/1
  Data Type Conversion3/1 -> Bitwise Operator4/1
  Data Type Conversion6/1 -> Bitwise Operator2/1
  Mux/1 -> "[v,w]"/1
  Bitwise Operator/1 -> Subsystem1/1(In1)
  Bitwise Operator6/1 -> Subsystem3/1(In1)
  Bitwise Operator7/1 -> Subsystem3/2(In2)
  Bitwise Operator4/1 -> Subsystem2/1(In1)
  Bitwise Operator5/1 -> Subsystem2/2(In2)
  Subsystem3/1(Output1) -> HTD/1
  Bitwise Operator3/1 -> Subsystem/1(In1)
  Bitwise Operator2/1 -> Subsystem/2(In2)
  Subsystem1/1(Output) -> HDD/1
  Subsystem2/1(Output) -> HTI/1
  Subsystem/1(Output) -> HDI/1

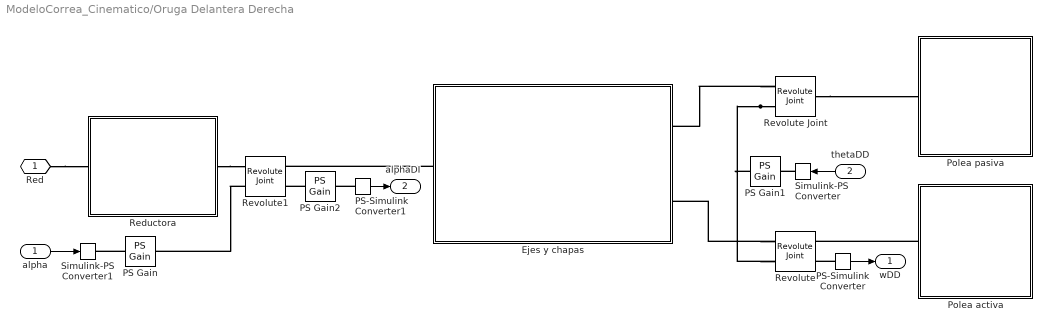
== system ModeloCorrea_Cinematico/Oruga Delantera Derecha ==
  alpha : Inport
  thetaDD : Inport  Port=2
  Ejes y chapas : Subsystem
      mask Display: image('Ejes y chapas.png');
  PS Gain : fl_lib/Physical Signals/Functions/PS Gain  gain=-1
  PS Gain1 : fl_lib/Physical Signals/Functions/PS Gain  gain=-1
  PS Gain2 : fl_lib/Physical Signals/Functions/PS Gain  gain=-1
  PS-Simulink Converter : nesl_utility/PS-Simulink Converter  PhysicalDomain=network_engine_domain  SubClassName=ps_output  LeftPortType=input  RightPortType=output  PseudoPeriodic=off  Frequencies=[]  VectorFormat=inherit  Unit=rad/s  AffineConversion=off
  PS-Simulink Converter1 : nesl_utility/PS-Simulink Converter  PhysicalDomain=network_engine_domain  SubClassName=ps_output  LeftPortType=input  RightPortType=output  PseudoPeriodic=off  Frequencies=[]  VectorFormat=inherit  Unit=rad  AffineConversion=off
  Polea activa : Subsystem
      mask Display: image('Polea activa.png');
  Polea pasiva : Subsystem
      mask Display: image('Polea pasiva.png');
  Reductora : Subsystem
      mask Display: image('Reductora.png');
  Revolute : sm_lib/Joints/Revolute Joint  JointMode=Normal  SenseConstraintForce=off  SenseConstraintForceX=off  SenseConstraintForceY=off  SenseConstraintForceZ=off  SenseConstraintTorque=off  SenseConstraintTorqueX=off  SenseConstraintTorqueY=off  SenseConstraintTorqueZ=off  SenseTotalForce=off  SenseTotalForceX=off  SenseTotalForceY=off  SenseTotalForceZ=off  SenseTotalTorque=off  SenseTotalTorqueX=off  SenseTotalTorqueY=off  SenseTotalTorqueZ=off  CompositeWrenchDir=FollowerOnBase  CompositeWrenchFrame=BaseFrame  EquilibriumPosition=0  EquilibriumPositionUnits=deg  SpringStiffness=0  SpringStiffnessUnits=N*m/deg  DampingCoefficient=5e-4  DampingCoefficientUnits=N*m/(deg/s)  TorqueActuationMode=ComputedTorque  MotionActuationMode=InputMotion  SensePosition=off  SenseVelocity=on  SenseAcceleration=off  SenseTorqueForce=off  SenseLowerLimitTorqueForce=off  SenseUpperLimitTorqueForce=off  LowerLimitSpecify=off  LowerLimitBound=-90  LowerLimitBoundUnits=deg  LowerLimitStiffness=1e4  LowerLimitStiffnessUnits=N*m/deg  LowerLimitDamping=10  LowerLimitDampingUnits=N*m/(deg/s)  LowerLimitTransitionRegionWidth=0.1  LowerLimitTransitionRegionWidthUnits=deg  UpperLimitSpecify=off  UpperLimitBound=90  UpperLimitBoundUnits=deg  UpperLimitStiffness=1e4  UpperLimitStiffnessUnits=N*m/deg  UpperLimitDamping=10  UpperLimitDampingUnits=N*m/(deg/s)  UpperLimitTransitionRegionWidth=0.1  UpperLimitTransitionRegionWidthUnits=deg  PositionTargetSpecify=on  PositionTargetPriority=Low  PositionTargetValue=smiData.RevoluteJoint(1).Rz.Pos  PositionTargetValueUnits=deg  VelocityTargetSpecify=off  VelocityTargetPriority=High  VelocityTargetValue=0  VelocityTargetValueUnits=deg/s
  Revolute Joint : sm_lib/Joints/Revolute Joint  JointMode=Normal  SenseConstraintForce=off  SenseConstraintForceX=off  SenseConstraintForceY=off  SenseConstraintForceZ=off  SenseConstraintTorque=off  SenseConstraintTorqueX=off  SenseConstraintTorqueY=off  SenseConstraintTorqueZ=off  SenseTotalForce=off  SenseTotalForceX=off  SenseTotalForceY=off  SenseTotalForceZ=off  SenseTotalTorque=off  SenseTotalTorqueX=off  SenseTotalTorqueY=off  SenseTotalTorqueZ=off  CompositeWrenchDir=FollowerOnBase  CompositeWrenchFrame=BaseFrame  EquilibriumPosition=0  EquilibriumPositionUnits=deg  SpringStiffness=0  SpringStiffnessUnits=N*m/deg  DampingCoefficient=5e-4  DampingCoefficientUnits=N*m/(deg/s)  TorqueActuationMode=ComputedTorque  MotionActuationMode=InputMotion  SensePosition=off  SenseVelocity=off  SenseAcceleration=off  SenseTorqueForce=off  SenseLowerLimitTorqueForce=off  SenseUpperLimitTorqueForce=off  LowerLimitSpecify=off  LowerLimitBound=-90  LowerLimitBoundUnits=deg  LowerLimitStiffness=1e4  LowerLimitStiffnessUnits=N*m/deg  LowerLimitDamping=10  LowerLimitDampingUnits=N*m/(deg/s)  LowerLimitTransitionRegionWidth=0.1  LowerLimitTransitionRegionWidthUnits=deg  UpperLimitSpecify=off  UpperLimitBound=90  UpperLimitBoundUnits=deg  UpperLimitStiffness=1e4  UpperLimitStiffnessUnits=N*m/deg  UpperLimitDamping=10  UpperLimitDampingUnits=N*m/(deg/s)  UpperLimitTransitionRegionWidth=0.1  UpperLimitTransitionRegionWidthUnits=deg  PositionTargetSpecify=off  PositionTargetPriority=High  PositionTargetValue=0  PositionTargetValueUnits=deg  VelocityTargetSpecify=off  VelocityTargetPriority=High  VelocityTargetValue=0  VelocityTargetValueUnits=deg/s
  Revolute1 : sm_lib/Joints/Revolute Joint  JointMode=Normal  SenseConstraintForce=off  SenseConstraintForceX=off  SenseConstraintForceY=off  SenseConstraintForceZ=off  SenseConstraintTorque=off  SenseConstraintTorqueX=off  SenseConstraintTorqueY=off  SenseConstraintTorqueZ=off  SenseTotalForce=off  SenseTotalForceX=off  SenseTotalForceY=off  SenseTotalForceZ=off  SenseTotalTorque=off  SenseTotalTorqueX=off  SenseTotalTorqueY=off  SenseTotalTorqueZ=off  CompositeWrenchDir=FollowerOnBase  CompositeWrenchFrame=BaseFrame  EquilibriumPosition=0  EquilibriumPositionUnits=deg  SpringStiffness=0  SpringStiffnessUnits=N*m/deg  DampingCoefficient=5e-4  DampingCoefficientUnits=N*m/(deg/s)  TorqueActuationMode=ComputedTorque  MotionActuationMode=InputMotion  SensePosition=on  SenseVelocity=off  SenseAcceleration=off  SenseTorqueForce=off  SenseLowerLimitTorqueForce=off  SenseUpperLimitTorqueForce=off  LowerLimitSpecify=on  LowerLimitBound=0  LowerLimitBoundUnits=deg  LowerLimitStiffness=1e4  LowerLimitStiffnessUnits=N*m/deg  LowerLimitDamping=10  LowerLimitDampingUnits=N*m/(deg/s)  LowerLimitTransitionRegionWidth=0.1  LowerLimitTransitionRegionWidthUnits=deg  UpperLimitSpecify=on  UpperLimitBound=90  UpperLimitBoundUnits=deg  UpperLimitStiffness=1e4  UpperLimitStiffnessUnits=N*m/deg  UpperLimitDamping=10  UpperLimitDampingUnits=N*m/(deg/s)  UpperLimitTransitionRegionWidth=0.1  UpperLimitTransitionRegionWidthUnits=deg  PositionTargetSpecify=on  PositionTargetPriority=Low  PositionTargetValue=smiData.RevoluteJoint(2).Rz.Pos  PositionTargetValueUnits=deg  VelocityTargetSpecify=off  VelocityTargetPriority=High  VelocityTargetValue=0  VelocityTargetValueUnits=deg/s
  Simulink-PS Converter : nesl_utility/Simulink-PS Converter  PhysicalDomain=network_engine_domain  SubClassName=ps_input  LeftPortType=input  RightPortType=output  PseudoPeriodic=off  Frequencies=[]  NoiseDistribution=none  NoiseParameters=[]  Unit=1  AffineConversion=off  FilteringAndDerivatives=filter  SimscapeFilterOrder=2  InputFilterTimeConstant=0.001  UdotUserProvided=0
  Simulink-PS Converter1 : nesl_utility/Simulink-PS Converter  PhysicalDomain=network_engine_domain  SubClassName=ps_input  LeftPortType=input  RightPortType=output  PseudoPeriodic=off  Frequencies=[]  NoiseDistribution=none  NoiseParameters=[]  Unit=1  AffineConversion=off  FilteringAndDerivatives=filter  SimscapeFilterOrder=2  InputFilterTimeConstant=0.001  UdotUserProvided=0
  Red : PMIOPort  Side=Left
  wDD : Outport
  alphaDI : Outport  Port=2
  wires:
  thetaDD/1 -> Simulink-PS Converter/1
  PS-Simulink Converter/1 -> wDD/1
  alpha/1 -> Simulink-PS Converter1/1
  PS-Simulink Converter1/1 -> alphaDI/1
  connections:
  Red/RConn1 -- Reductora/LConn1
  Ejes y chapas/LConn1 -- Revolute1/RConn1
  Reductora/RConn1 -- Revolute1/LConn1
  Polea activa/LConn1 -- Revolute/RConn1
  Revolute/LConn1 -- Ejes y chapas/RConn2
  Revolute Joint/RConn1 -- Polea pasiva/LConn1
  Revolute Joint/LConn1 -- Ejes y chapas/RConn1
  Revolute1/LConn2 -- PS Gain/RConn1
  Revolute Joint/LConn2 -- PS Gain1/RConn1 -- Revolute/LConn2
  PS-Simulink Converter/LConn1 -- Revolute/RConn2
  PS-Simulink Converter1/LConn1 -- PS Gain2/RConn1
  PS Gain/LConn1 -- Simulink-PS Converter1/RConn1
  Simulink-PS Converter/RConn1 -- PS Gain1/LConn1
  PS Gain2/LConn1 -- Revolute1/RConn2
